simulink model "AirFilter_harness"  (Simulink 7.7)
settings: Solver=FixedStepDiscrete  SolverMode=SingleTasking  StartTime=0.0  StopTime=100  FixedStep=0.1  RelTol=1e-3
InitFcn:
  | if signalbuilder('AirFilter_harness/Signal_Builder','activegroup') == 3
  |   CD_AIR_FILTER_FUNCTION.DataType = 'uint8';
  |   CD_AIR_FILTER_FUNCTION.Value = 255;
  | else
  |   CD_AIR_FILTER_FUNCTION.DataType = 'uint8';
  |   CD_AIR_FILTER_FUNCTION.Value = 0;
  | end
  | 
  | if signalbuilder('AirFilter_harness/Signal_Builder','activegroup') == 4
  |   CD_ECU_FUNCTION.DataType = 'uint8';
  |   CD_ECU_FUNCTION.Value = 0;
  | else
  |   CD_ECU_FUNCTION.DataType = 'uint8';
  |   CD_ECU_FUNCTION.Value = 255;
  | end
  | 
  | CD_AIR_FILTER_DEBOUNCE_NOT_CONNECTED.DataType = 'uint16';
  | CD_AIR_FILTER_DEBOUNCE_NOT_CONNECTED.Value = 100;
  | 
  | 
  | CD_AIR_FILTER_DEBOUNCE_PLUGGED.DataType = 'uint16';
  | CD_AIR_FILTER_DEBOUNCE_PLUGGED.Value = 70;
  | 
  | 
  | CD_AIR_FILTER_DEBOUNCE_NORMAL.DataType = 'uint16';
  | CD_AIR_FILTER_DEBOUNCE_NORMAL.Value = 50;
undefined symbols (not defined in the file): ACTIVE, ENGINE_NOT_RUNNING, ENGINE_RUNNING, INACTIVE, NON_FUNCTIONAL, NORMAL, NOT_CONNECTED, PLUGGED, sigbuilder_block, srate100
CloseFcn:
  | rtwprivate ssgencode ModelCloseRequest sle_main_controller
settings Model: Creator=smindema  LastModifiedBy=aliebel  RecordCoverage=on  CovMetricSettings=dcw  CovHTMLOptions=-aTS=1 -bRG=1 -bTC=1 -hTR=0 -nFC=0 -scm=1 -bcm=1 -xEv=0  CovCumulativeReport=on
settings MATStruct: SampleTime=0.01  Offset=0  Priority=[1.0]
settings DataIOCC: LimitDataPoints=off  SaveOutput=off  SaveTime=off
settings OptimizationCC: BlockReduction=off  InlineParams=on  ExpressionFolding=off  StateBitsets=on  DataBitsets=on  UseTempVars=on  InitFltsAndDblsToZero=on  NoFixptDivByZeroProtection=on  EfficientFloat2IntCast=on  OptimizeModelRefInitCode=on
settings DebuggingCC: SaveWithParameterizedLinksMsg=none  MultiTaskDSMMsg=warning  MultiTaskCondExecSysMsg=none  IntegerOverflowMsg=none  ModelReferenceCSMismatchMessage=warning
settings HardwareCC: ProdBitPerInt=16  ProdBitPerPointer=16  ProdIntDivRoundTo=Floor  ProdEndianess=BigEndian  ProdWordSize=16  ProdHWDeviceType=Motorola HC12
settings ModelReferenceCC: ModelReferenceNumInstancesAllowed=Single
settings SFSimCC: SimCustomHeaderCode="#include \"SendMsgNow.h\""  SimUserSources=SendMsgNow_Blank.c  SimUserIncludeDirs=functions
settings RTWCC: SystemTargetFile=ert.tlc  GenCodeOnly=on  TemplateMakefile=ert_default_tmf  Description=Real-Time Workshop Embedded Coder (no auto configuration)  GenerateReport=on  RetainRTWFile=on  ProcessScript=ert_make_rtw_hook  IncludeHyperlinkInReport=on  LaunchReport=on  IncludeERTFirstTime=on
settings RTWCC: CustomHeaderCode=|
  | #include "cpp_req_defines.h"
  | #include "hw_fin.h"
  | #include "cdata.h"
settings CodeAppCC: IgnoreCustomStorageClasses=off  DefineNamingRule=UpperCase
settings ERTTargetCC: TargetFcnLib=ansi_tfl_tmw.mat  FunctionExecutionProfile=off  MultiwordLength=2048  GenerateSampleERTMain=on  IncludeMdlTerminateFcn=off  SupportAbsoluteTime=off  SupportNonFinite=off  SupportComplex=off  PurelyIntegerCode=on  ERTCustomFileTemplate=gen_rtw_req_defines_h.tlc  GlobalDataDefinition=InSeparateSourceFile  GlobalDataReference=InSeparateHeaderFile  ConvertIfToSwitch=off

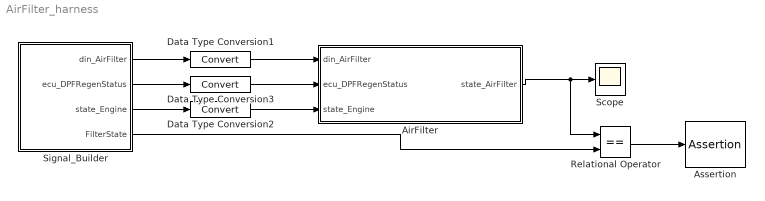
== system AirFilter_harness ==
  AirFilter : Subsystem  TreatAsAtomicUnit=on  SystemSampleTime=srate100  RTWFileName=mod_Inputs
      settings: RTWSystemCode=Function  RTWFileNameOpts=User specified
  Assertion : Assertion  Enabled=off
  Data Type Conversion1 : DataTypeConversion
  Data Type Conversion2 : DataTypeConversion
  Data Type Conversion3 : DataTypeConversion
  Relational Operator : RelationalOperator  Operator===  OutDataTypeStr=boolean
  Scope : Scope
      settings: TimeRange=100  YMin=0  YMax=20  MaxDataPoints=100000
  Signal_Builder : Subsystem  Tag=STV Subsys  RequirementInfo={'other' '' '' 'true' 'Test not connected error' '' ; 'other' '' '' 'true' 'Test plugged filter error' '' ; 'other' '' '' 'true' 'Test setting input to nonfunctional' '' } %GIDa_49457480_5376_4aab_abc2_8675615ddb40  LoadFcn=sigbuilder_block('load',[524.25 371.25 627 415.5 ]);  StartFcn=sigbuilder_block('start');  StopFcn=sigbuilder_block('stop');  ClipboardFcn=sigbuilder_block('clipboard');  mask(Sigbuilder block){}
      mask help: Sigbuilder GUI
      mask init:
      | if ~strcmp(get_param(bdroot(gcbh),'SimulationStatus'),'stopped') tuvar = sigbuilder_block('maskInit'); end
      settings: CopyFcn=sigbuilder_block('copy');  DeleteFcn=sigbuilder_block('delete');  ModelCloseFcn=sigbuilder_block('modelClose');  PreSaveFcn=sigbuilder_block('preSave');  NameChangeFcn=sigbuilder_block('namechange');  OpenFcn=sigbuilder_block('open',[660.75 177 627 415.5 ]);  CloseFcn=sigbuilder_block('close');
      mask Display: plot(0,0,100,100,[10,10,40,40,10],[80,20,20,80,80],[40,10],[50,50], [40,27,10],[65,72,56],[40,25,25,10],[28,28,43,43]);
  wires:
  Signal_Builder/1(din_AirFilter) -> Data Type Conversion1/1
  Signal_Builder/3(state_Engine) -> Data Type Conversion2/1
  Data Type Conversion1/1 -> AirFilter/1(din_AirFilter)
  Data Type Conversion2/1 -> AirFilter/3(state_Engine)
  AirFilter/1(state_AirFilter) -> Scope/1, Relational Operator/1
  Signal_Builder/4(FilterState) -> Relational Operator/2
  Relational Operator/1 -> Assertion/1
  Signal_Builder/2(ecu_DPFRegenStatus) -> Data Type Conversion3/1
  Data Type Conversion3/1 -> AirFilter/2(ecu_DPFRegenStatus)

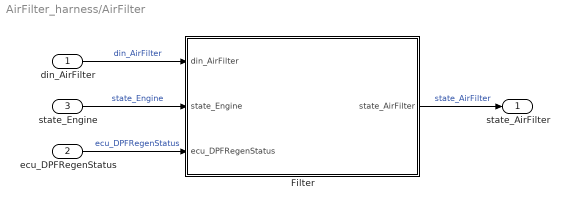
== system AirFilter_harness/AirFilter ==
  din_AirFilter : Inport  OutDataTypeStr=uint8
  ecu_DPFRegenStatus : Inport  Port=2  OutDataTypeStr=uint8
  state_Engine : Inport  Port=3  OutDataTypeStr=uint8
  Filter : Stateflow chart  TreatAsAtomicUnit=on
  state_AirFilter : Outport  OutDataTypeStr=uint8
  wires:
  Filter/1(state_AirFilter) -> state_AirFilter/1  "state_AirFilter"
  state_Engine/1 -> Filter/2(state_Engine)  "state_Engine"
  din_AirFilter/1 -> Filter/1(din_AirFilter)  "din_AirFilter"
  ecu_DPFRegenStatus/1 -> Filter/3(ecu_DPFRegenStatus)  "ecu_DPFRegenStatus"

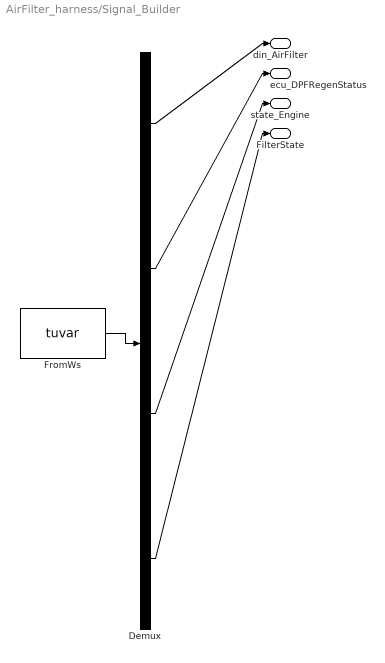
== system AirFilter_harness/Signal_Builder ==
  Demux : Demux  Tag=STV Demux
  FromWs : FromWorkspace  Tag=STV FromWs  VariableName=tuvar  SampleTime=0  SigBuilderData=DataTag0  VnvData=DataTag1
      SigBuilderData=|
      | common.afterFinalStr = 'Extrapolate'
      | common.sampleTime = 0
      | dataSet(1).timeRange = [0 100]
      | dataSet(1).name = 'Not Connected'
      | dataSet(2).timeRange = [0 100]
      | dataSet(2).name = 'Plugged'
      | dataSet(3).timeRange = [0 100]
      | dataSet(3).name = 'NonFunctional'
      | dataSet(4).timeRange = [0 100]
      | dataSet(4).name = 'ECU'
      | sbobj.Groups(1).Name = 'Not Connected'
      | sbobj.Groups(1).Signals(1).Name = 'din_AirFilter'
      | sbobj.Groups(1).Signals(1).XData = [0 1 1 2.99 2.99 4 4 6.02 6.02 20.4 20.4 27.8 27.8 30 30 61.6 61.6 62.6 62.6 70 70 87.8 87.8 92 92 100]
      | sbobj.Groups(1).Signals(1).YData = [0 0 1 1 0 0 1 1 0 0 1 1 0 0 1 1 0 0 1 1 0 0 1 1 0 0]
      | sbobj.Groups(1).Signals(2).Name = 'ecu_DPFRegenStatus'
      | sbobj.Groups(1).Signals(2).XData = [0 100]
      | sbobj.Groups(1).Signals(2).YData = [0 0]
      | sbobj.Groups(1).Signals(3).Name = 'state_Engine'
      | sbobj.Groups(1).Signals(3).XData = [0 60.2 60.2 80.2 80.2 100]
      | sbobj.Groups(1).Signals(3).YData = [1 1 3 3 2 2]
      | sbobj.Groups(1).Signals(4).Name = 'FilterState'
      | sbobj.Groups(1).Signals(4).XData = [0 40.1 40.1 75.1 75.1 100]
      | sbobj.Groups(1).Signals(4).YData = [8 8 16 16 8 8]
      | sbobj.Groups(2).Name = 'Plugged'
      | sbobj.Groups(2).Signals(1).Name = 'din_AirFilter'
      | sbobj.Groups(2).Signals(1).XData = [0 1 1 1.99 1.99 4 4 5.01 5.01 20.4 20.4 26.6 26.6 28.2 28.2 70 70 100]
      | sbobj.Groups(2).Signals(1).YData = [0 0 1 1 0 0 1 1 0 0 1 1 0 0 1 1 0 0]
      | sbobj.Groups(2).Signals(2).Name = 'ecu_DPFRegenStatus'
      | sbobj.Groups(2).Signals(2).XData = [0 23.2 23.2 100]
      | sbobj.Groups(2).Signals(2).YData = [0 0 1 1]
      | sbobj.Groups(2).Signals(3).Name = 'state_Engine'
      | sbobj.Groups(2).Signals(3).XData = [0 59.2 59.2 100]
      | sbobj.Groups(2).Signals(3).YData = [3 3 1 1]
      | sbobj.Groups(2).Signals(4).Name = 'FilterState'
      | sbobj.Groups(2).Signals(4).XData = [0 35.3 35.3 100]
      | sbobj.Groups(2).Signals(4).YData = [8 8 17 17]
      | sbobj.Groups(3).Name = 'NonFunctional'
      | sbobj.Groups(3).Signals(1).Name = 'din_AirFilter'
      | sbobj.Groups(3).Signals(1).XData = [0 1 1 2.6 2.99 2.99 4 4 6.02 6.02 20.4 20.4 28 28 29 29 70 70 100]
      | sbobj.Groups(3).Signals(1).YData = [0 0 1 1 1 0 0 1 1 0 0 1 1 0 0 1 1 0 0]
      | sbobj.Groups(3).Signals(2).Name = 'ecu_DPFRegenStatus'
      | sbobj.Groups(3).Signals(2).XData = [0 100]
      | sbobj.Groups(3).Signals(2).YData = [0 0]
      | sbobj.Groups(3).Signals(3).Name = 'state_Engine'
      | sbobj.Groups(3).Signals(3).XData = [0 59.8 59.8 100]
      | sbobj.Groups(3).Signals(3).YData = [1 1 3 3]
      | sbobj.Groups(3).Signals(4).Name = 'FilterState'
      | sbobj.Groups(3).Signals(4).XData = [0 100]
      | sbobj.Groups(3).Signals(4).YData = [8 8]
      | sbobj.Groups(4).Name = 'ECU'
      | sbobj.Groups(4).Signals(1).Name = 'din_AirFilter'
      | sbobj.Groups(4).Signals(1).XData = [0 1 1 2.6 2.99 2.99 4 4 6.02 6.02 20.4 28 60 60 84.8 84.8 100]
      | sbobj.Groups(4).Signals(1).YData = [0 0 1 1 1 0 0 1 1 0 0 0 0 1 1 0 0]
      | sbobj.Groups(4).Signals(2).Name = 'ecu_DPFRegenStatus'
      | sbobj.Groups(4).Signals(2).XData = [0 57.2 57.2 66 66 100]
      | sbobj.Groups(4).Signals(2).YData = [0 0 1 1 0 0]
      | sbobj.Groups(4).Signals(3).Name = 'state_Engine'
      | sbobj.Groups(4).Signals(3).XData = [0 59.8 59.8 100]
      | sbobj.Groups(4).Signals(3).YData = [1 1 3 3]
      | sbobj.Groups(4).Signals(4).Name = 'FilterState'
      | sbobj.Groups(4).Signals(4).XData = [0 100]
      | sbobj.Groups(4).Signals(4).YData = [8 8]
  din_AirFilter : Outport  Tag=STV Outport
  ecu_DPFRegenStatus : Outport  Tag=STV Outport  Port=2
  state_Engine : Outport  Tag=STV Outport  Port=3
  FilterState : Outport  Tag=STV Outport  Port=4
  wires:
  FromWs/1 -> Demux/1
  Demux/1 -> din_AirFilter/1
  Demux/2 -> ecu_DPFRegenStatus/1
  Demux/3 -> state_Engine/1
  Demux/4 -> FilterState/1

== stateflow chart AirFilter/Filter ==
  state PLUGGED
    state DEBOUNCE
      en:debounceCount = 0;
      du:debounceCount++;
    state PLUGGED
      en:state_AirFilter = PLUGGED;
    (default) -> PLUGGED.DEBOUNCE
    PLUGGED.DEBOUNCE -> PLUGGED.PLUGGED : [(debounceCount >= CD_AIR_FILTER_DEBOUNCE_PLUGGED)]
  state NORMAL
    state DEBOUNCE
      en:debounceCount = 0;
      du:debounceCount++;
    state NORMAL
      en:state_AirFilter = NORMAL;
    (default) -> NORMAL.DEBOUNCE
    NORMAL.DEBOUNCE -> NORMAL.NORMAL : [(debounceCount >= CD_AIR_FILTER_DEBOUNCE_NORMAL)...
        | || (state_AirFilter == NORMAL)]
  state NON_FUNCTIONAL
    en:state_AirFilter = NORMAL;
  state NOT_CONNECTED
    state DEBOUNCE
      en:debounceCount = 0;
      du:debounceCount++;
    state NOT_CONNECTED
      en:state_AirFilter = NOT_CONNECTED;
    (default) -> NOT_CONNECTED.DEBOUNCE
    NOT_CONNECTED.DEBOUNCE -> NOT_CONNECTED.NOT_CONNECTED : [(debounceCount >= CD_AIR_FILTER_DEBOUNCE_NOT_CONNECTED)...
        | || (state_AirFilter == NOT_CONNECTED)]
  (default) -> NON_FUNCTIONAL
  PLUGGED -> NORMAL : [(din_AirFilter != ACTIVE)...
      | && (state_AirFilter == NORMAL)]
  NON_FUNCTIONAL -> NORMAL : [(CD_AIR_FILTER_FUNCTION != NON_FUNCTIONAL)]
  NORMAL -> PLUGGED [order 1] : [(din_AirFilter == ACTIVE)...
      | && (state_Engine == ENGINE_RUNNING)...
      | && (state_AirFilter != NOT_CONNECTED)...
      | && ((CD_ECU_FUNCTION == NON_FUNCTIONAL)...
      |       || ((CD_ECU_FUNCTION != NON_FUNCTIONAL) && (ecu_DPFRegenStatus == INACTIVE)))]
  NORMAL -> NOT_CONNECTED [order 2] : [(din_AirFilter == ACTIVE)...
      | && ((state_Engine == ENGINE_NOT_RUNNING) || (state_AirFilter == NOT_CONNECTED))]
  NOT_CONNECTED -> NORMAL : [(din_AirFilter != ACTIVE)]
  data: din_AirFilter input uint8; state_Engine input uint8; state_AirFilter output uint8; CD_AIR_FILTER_DEBOUNCE_NORMAL parameter uint16; CD_AIR_FILTER_DEBOUNCE_NOT_CONNECTED parameter uint16; CD_AIR_FILTER_DEBOUNCE_PLUGGED parameter uint16; CD_AIR_FILTER_FUNCTION parameter uint8; debounceCount local uint16 =0; ACTIVE parameter uint8 =1; ENGINE_NOT_RUNNING parameter uint8 =1; PLUGGED parameter uint8 =17; NON_FUNCTIONAL parameter uint8 =255; ENGINE_RUNNING parameter uint8 =3; NORMAL parameter uint8 =8; NOT_CONNECTED parameter uint8 =17; CD_ECU_FUNCTION parameter uint8; ecu_DPFRegenStatus input uint8; INACTIVE parameter uint8
